simulink model "FmTxRx"  (R2015b)
settings: Solver=VariableStepAuto  StartTime=0.0  StopTime=10.0  RelTol=1e-3
undefined symbols (not defined in the file): SLIF_fc_IM, SLIF_fc_IMDS, SLIF_fc_IMDT, SLIF_fc_LO, SLIF_fc_RF, SLIF_Frame, SLIF_ModIndex, SLIF_PSF_SampPerSym, SLIF_Rsymbol
libraries: dspmathops x8, simrfV2elements x7, dspstat3 x7, simrfV2util1 x6, dspsrcs4 x4, commrflib2 x4, commrandsrc2 x3, commobslib x3, commdigbbndfm2 x3, dspvision x1, dspsnks4 x1
settings Model: Creator=dominikguz  LastModifiedBy=dominikguz

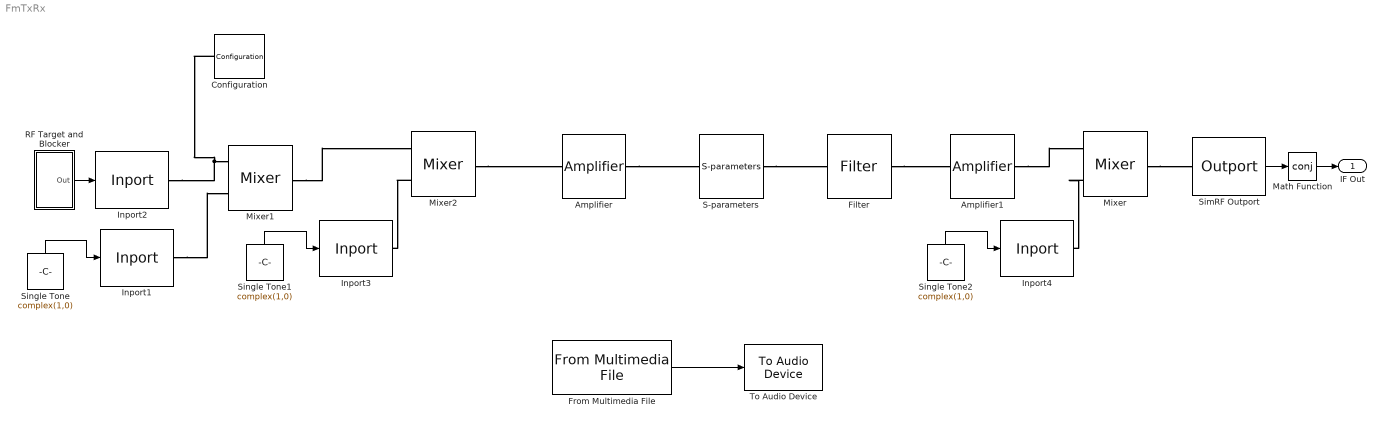
== system FmTxRx ==
  Amplifier : simrfV2elements/Amplifier  classname=amplifier  DataSource=Data file  File=simrfV2_unitygain.s2p  Paramtype=S-parameters  Sparam=[0 0;1 0]  SparamFreq=1e9 Hz  SparamZ0=50  Residues=0  Poles=0  DF={0 0; 1 0}  Source_linear_gain=Available power gain  linear_gain=10 dB  Zin=50  Zout=50  Source_Poly=Even and odd order  Poly_Coeffs=[0 1]  IPType=Output  IP2=inf dBm  IP3=inf dBm  P1dB=inf dBm  Psat=inf dBm  Gcomp=inf dBm  NF=0  InternalGrounding=on  SourceFreq=Extracted from data source  PlotFreq=[1e9:1e6:3e9] Hz  PlotType=X-Y plane  YParam1=S11  YFormat1=Magnitude (decibels)  YParam2=None  YFormat2=Magnitude (decibels)  YOption=Linear  XOption=Linear  SparamRepresentation=Time domain (rationalfit)  FitTol=-40  FitOpt=Fit individually  AutoImpulseLength=on  ImpulseLength=1e-10 s
  Amplifier1 : simrfV2elements/Amplifier  classname=amplifier  DataSource=Data file  File=simrfV2_unitygain.s2p  Paramtype=S-parameters  Sparam=[0 0;1 0]  SparamFreq=1e9 Hz  SparamZ0=50  Residues=0  Poles=0  DF={0 0; 1 0}  Source_linear_gain=Available power gain  linear_gain=10 dB  Zin=50  Zout=50  Source_Poly=Even and odd order  Poly_Coeffs=[0 1]  IPType=Output  IP2=inf dBm  IP3=inf dBm  P1dB=inf dBm  Psat=inf dBm  Gcomp=inf dBm  NF=0  InternalGrounding=on  SourceFreq=Extracted from data source  PlotFreq=[1e9:1e6:3e9] Hz  PlotType=X-Y plane  YParam1=S11  YFormat1=Magnitude (decibels)  YParam2=None  YFormat2=Magnitude (decibels)  YOption=Linear  XOption=Linear  SparamRepresentation=Time domain (rationalfit)  FitTol=-40  FitOpt=Fit individually  AutoImpulseLength=on  ImpulseLength=1e-10 s
  Configuration : simrfV2util1/Configuration  AutoFreq=on  Tones=[] Hz  Harmonics=[]  NormalizeCarrierPower=on  SolverType=Auto  StepSize=1e-6 s  AddNoise=on  Temperature=290.0 K  SolverDelFlag=0
  Filter : simrfV2elements/Filter  classname=filter  DesignMethod=Butterworth  ResponseType=Lowpass  Implementation=LC Tee  UseFilterOrder=on  FilterOrder=3  PassFreq_lp=1 GHz  PassFreq_hp=2 GHz  PassFreq_bp=[2 3] GHz  PassFreq_bs=[1 4] GHz  PassAtten=10*log10(2)  StopFreq_lp=2 GHz  StopFreq_hp=1 GHz  StopFreq_bp=[1.5 3.5] GHz  StopFreq_bs=[2.1 2.9] GHz  StopAtten=40  Rsrc=50  Rload=50  InternalGrounding=on  PlotFuncLeft=Voltage transfer  PlotLeftForm=Magnitude (decibels)  PlotRightOnVT=None  PlotRightNoTD=None  PlotRightNoGD=None  PlotRightNoIR=None  PlotRightNoSR=None  PlotRightForm=Magnitude (decibels)  FreqPoints=logspace(0,10,101)  Freq_unit=Hz  TimePoints=linspace(0,1,1e6+1)  Time_unit=s  XaxisScale=Linear  YaxisScale=Linear
  From Multimedia File : dspvision/From Multimedia File  inputFilename=speech_dft.mp3  loop=on  numPlays=inf  outputStreams=Audio only  videoDataType=single  audioDataType=double  inheritSampleTime=on  userDefinedSampleTime=1/30  noAudioOutput=off  isIntensityVideo=off  fourcc=RGB  colorVideoFormat=Separate color signals  outputEOF=off  dataOrg=Column-major  audioFrameSize=1024  computeAudioFrameSize=off  outSamplingMode=Sample based
  Inport1 : simrfV2util1/Inport  SimulinkInputSignalType=Ideal voltage  CarrierFreq=[SLIF_fc_LO] Hz  ZS=0  InternalGrounding=on
  Inport2 : simrfV2util1/Inport  SimulinkInputSignalType=Ideal voltage  CarrierFreq=[SLIF_fc_RF,SLIF_fc_IM,SLIF_fc_IMDS,SLIF_fc_IMDT] Hz  ZS=0  InternalGrounding=on
  Inport3 : simrfV2util1/Inport  SimulinkInputSignalType=Ideal voltage  CarrierFreq=[SLIF_fc_LO] Hz  ZS=0  InternalGrounding=on
  Inport4 : simrfV2util1/Inport  SimulinkInputSignalType=Ideal voltage  CarrierFreq=[SLIF_fc_LO] Hz  ZS=0  InternalGrounding=on
  Math Function : Math  Operator=conj  SaturateOnIntegerOverflow=on
  Mixer : simrfV2elements/Mixer  classname=mixer  Source_linear_gain=Available power gain  linear_gain=0 dB  Zin=50  Zout=50  ZLO=inf  Source_Poly=Even and odd order  Poly_Coeffs=[0 1]  IPType=Output  IP2=Inf dBm  IP3=Inf dBm  P1dB=Inf dBm  Psat=Inf dBm  Gcomp=Inf dBm  NF=0  InternalGrounding=on
  Mixer1 : simrfV2elements/Mixer  classname=mixer  Source_linear_gain=Available power gain  linear_gain=0 dB  Zin=50  Zout=50  ZLO=inf  Source_Poly=Even and odd order  Poly_Coeffs=[0 1]  IPType=Output  IP2=Inf dBm  IP3=Inf dBm  P1dB=Inf dBm  Psat=Inf dBm  Gcomp=Inf dBm  NF=0  InternalGrounding=on
  Mixer2 : simrfV2elements/Mixer  classname=mixer  Source_linear_gain=Available power gain  linear_gain=0 dB  Zin=50  Zout=50  ZLO=inf  Source_Poly=Even and odd order  Poly_Coeffs=[0 1]  IPType=Output  IP2=Inf dBm  IP3=Inf dBm  P1dB=Inf dBm  Psat=Inf dBm  Gcomp=Inf dBm  NF=0  InternalGrounding=on
  RF Target and Blocker : Subsystem
  S-parameters : simrfV2elements/S-parameters  classname=sparam_element  DataSource=Data file  File=simrfV2_unitygain.s2p  Paramtype=S-parameters  Sparam=[0 0;1 0]  SparamFreq=1e9 Hz  SparamZ0=50  Residues=0  Poles=0  DF={0 0; 1 0}  FitOpt=Share all poles  FitTol=-40  SourceFreq=Extracted from data source  PlotFreq=[1e9:1e6:3e9] Hz  PlotType=X-Y plane  YParam1=S11  YFormat1=Magnitude (decibels)  YParam2=None  YFormat2=Magnitude (decibels)  YOption=Linear  XOption=Linear  AddNoise=off  InternalGrounding=on  SparamRepresentation=Time domain (rationalfit)  AutoImpulseLength=on  ImpulseLength=1e-10 s
  SimRF Outport : simrfV2util1/Outport  SensorType=Ideal voltage  OutputFormat=Complex Baseband  CarrierFreq=SLIF_fc_IF Hz  ZL=Inf  InternalGrounding=on  StepSize=-1 s  AutoStep=off
  Single Tone : Constant  Value=complex(1,0)
  Single Tone1 : Constant  Value=complex(1,0)
  Single Tone2 : Constant  Value=complex(1,0)
  To Audio Device : dspsnks4/To Audio Device  deviceName=Default  inheritSampleRate=on  sampleRate=44100  deviceDatatype=Determine from input data type  autoBufferSize=on  bufferSize=4096  queueDuration=1.0  defaultOutputChannelMapping=on  outputChannelMapping=1:2  outputNumUnderrunSamples=off
  IF Out : Outport
  wires:
  From Multimedia File/1 -> To Audio Device/1
  SimRF Outport/1 -> Math Function/1
  Math Function/1 -> IF Out/1
  RF Target and Blocker/1(Out) -> Inport2/1
  Single Tone/1 -> Inport1/1
  Single Tone1/1 -> Inport3/1
  Single Tone2/1 -> Inport4/1
  connections:
  Filter/RConn1 -- Amplifier1/LConn1
  S-parameters/RConn1 -- Filter/LConn1
  Amplifier/RConn1 -- S-parameters/LConn1
  Mixer2/RConn1 -- Amplifier/LConn1
  Mixer1/RConn1 -- Mixer2/LConn1
  Amplifier1/RConn1 -- Mixer/LConn1
  Configuration/LConn1 -- Inport2/RConn1 -- Mixer1/LConn1
  Mixer/RConn1 -- SimRF Outport/LConn1
  Inport1/RConn1 -- Mixer1/LConn2
  Mixer2/LConn2 -- Inport3/RConn1
  Mixer/LConn2 -- Inport4/RConn1

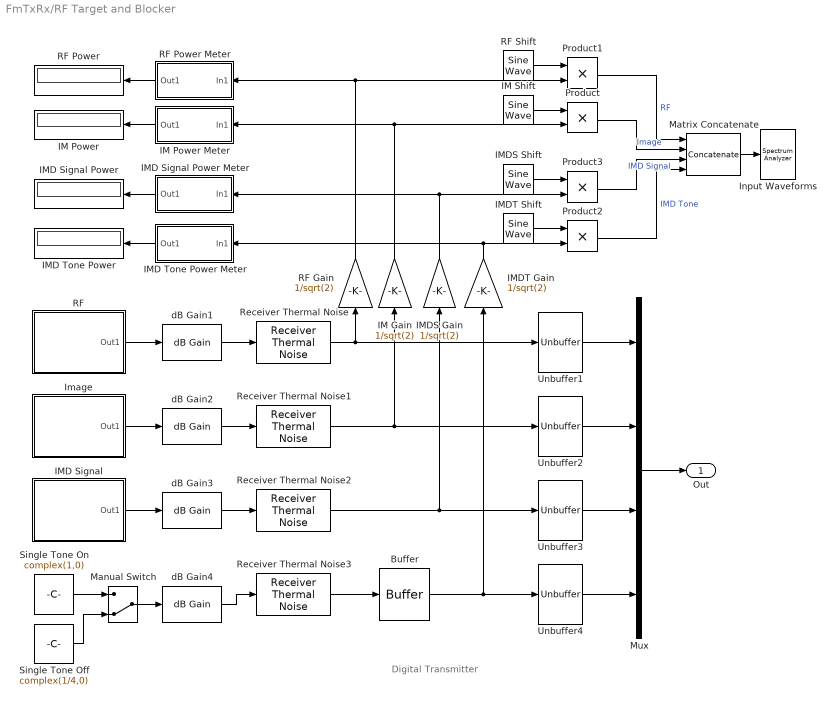
== system FmTxRx/RF Target and Blocker ==
  note: Digital Transmitter
  Buffer : Buffer  N=SLIF_PSF_SampPerSym*SLIF_Frame  TreatMby1Signals=One channel
  IM Gain : Gain  Gain=1/sqrt(2)
  IM Power : Display
  IM Power Meter : Subsystem
  IM Shift : dspsrcs4/Sine Wave  Amplitude=2  Frequency=SLIF_fc_LO-SLIF_fc_RF  Phase=0  SampleMode=Discrete  OutComplex=Complex  CompMethod=Trigonometric fcn  TableSize=Speed  SampleTime=1/(SLIF_Rsymbol*SLIF_PSF_SampPerSym)  SamplesPerFrame=SLIF_PSF_SampPerSym*SLIF_Frame  ResetState=Restart at time zero  OutputFrames=on  dataType=double  wordLen=16  udDataType=sfix(16)  fracBitsMode=Best precision  numFracBits=15  OutDataTypeStr=double  LastOutDataTypeStr=double
  IMD Signal : Subsystem
  IMD Signal Power : Display
  IMD Signal Power Meter : Subsystem
  IMD Tone Power : Display
  IMD Tone Power Meter : Subsystem
  IMDS Gain : Gain  Gain=1/sqrt(2)
  IMDS Shift : dspsrcs4/Sine Wave  Amplitude=2  Frequency=SLIF_fc_IMDS-SLIF_fc_RF  Phase=0  SampleMode=Discrete  OutComplex=Complex  CompMethod=Trigonometric fcn  TableSize=Speed  SampleTime=1/(SLIF_Rsymbol*SLIF_PSF_SampPerSym)  SamplesPerFrame=SLIF_PSF_SampPerSym*SLIF_Frame  ResetState=Restart at time zero  OutputFrames=on  dataType=double  wordLen=16  udDataType=sfix(16)  fracBitsMode=Best precision  numFracBits=15  OutDataTypeStr=double  LastOutDataTypeStr=double
  IMDT Gain : Gain  Gain=1/sqrt(2)
  IMDT Shift : dspsrcs4/Sine Wave  Amplitude=2  Frequency=SLIF_fc_IMDT-SLIF_fc_RF  Phase=0  SampleMode=Discrete  OutComplex=Complex  CompMethod=Trigonometric fcn  TableSize=Speed  SampleTime=1/(SLIF_Rsymbol*SLIF_PSF_SampPerSym)  SamplesPerFrame=SLIF_PSF_SampPerSym*SLIF_Frame  ResetState=Restart at time zero  OutputFrames=on  dataType=double  wordLen=16  udDataType=sfix(16)  fracBitsMode=Best precision  numFracBits=15  OutDataTypeStr=double  LastOutDataTypeStr=double
  Image : Subsystem
  Input Waveforms : SpectrumAnalyzer
  Manual Switch : ManualSwitch  CurrentSetting=0
  Matrix Concatenate : Concatenate  NumInputs=4  Mode=Multidimensional array  ConcatenateDimension=2
  Mux : Mux
  Product{,1..3} (4 alike) : Product  RndMeth=Zero
  RF : Subsystem
  RF Gain : Gain  Gain=1/sqrt(2)
  RF Power : Display
  RF Power Meter : Subsystem
  RF Shift : dspsrcs4/Sine Wave  Amplitude=2  Frequency=0  Phase=0  SampleMode=Discrete  OutComplex=Complex  CompMethod=Trigonometric fcn  TableSize=Speed  SampleTime=1/(SLIF_Rsymbol*SLIF_PSF_SampPerSym)  SamplesPerFrame=SLIF_PSF_SampPerSym*SLIF_Frame  ResetState=Restart at time zero  OutputFrames=on  dataType=double  wordLen=16  udDataType=sfix(16)  fracBitsMode=Best precision  numFracBits=15  OutDataTypeStr=double  LastOutDataTypeStr=double
  Receiver Thermal Noise{,1..3} (4 alike) : commrflib2/Receiver Thermal Noise  method=Noise temperature  ntemp=293  nfigure=3.01  nfactor=2  seed=67987
  Single Tone Off : Constant  Value=complex(1/4,0)
  Single Tone On : Constant  Value=complex(1,0)
  Unbuffer{1..4} (4 alike) : Unbuffer  SampleBasedProcessing=Same as frame based
  dB Gain1 : dspmathops/dB Gain  dB=-97  intype=Amplitude
  dB Gain2 : dspmathops/dB Gain  dB=-67  intype=Amplitude
  dB Gain3 : dspmathops/dB Gain  dB=-60  intype=Amplitude
  dB Gain4 : dspmathops/dB Gain  dB=-60  intype=Amplitude
  Out : Outport
  wires:
  Mux/1 -> Out/1
  RF Power Meter/1(Out1) -> RF Power/1
  IM Power Meter/1(Out1) -> IM Power/1
  Matrix Concatenate/1 -> Input Waveforms/1
  Image/1(Out1) -> dB Gain2/1
  RF/1(Out1) -> dB Gain1/1
  dB Gain1/1 -> Receiver Thermal Noise/1
  Receiver Thermal Noise/1 -> Unbuffer1/1, RF Gain/1
  dB Gain2/1 -> Receiver Thermal Noise1/1
  Receiver Thermal Noise1/1 -> Unbuffer2/1, IM Gain/1
  IM Shift/1 -> Product/1
  RF Shift/1 -> Product1/1
  Product1/1 -> Matrix Concatenate/1  "RF"
  IMD Signal/1(Out1) -> dB Gain3/1
  dB Gain3/1 -> Receiver Thermal Noise2/1
  Receiver Thermal Noise2/1 -> Unbuffer3/1, IMDS Gain/1
  IMD Signal Power Meter/1(Out1) -> IMD Signal Power/1
  dB Gain4/1 -> Receiver Thermal Noise3/1
  Receiver Thermal Noise3/1 -> Buffer/1
  IMD Tone Power Meter/1(Out1) -> IMD Tone Power/1
  IMDS Shift/1 -> Product3/1
  IMDT Shift/1 -> Product2/1
  Product3/1 -> Matrix Concatenate/3  "IMD Signal"
  Product2/1 -> Matrix Concatenate/4  "IMD Tone"
  Single Tone On/1 -> Manual Switch/1
  Single Tone Off/1 -> Manual Switch/2
  Manual Switch/1 -> dB Gain4/1
  Unbuffer4/1 -> Mux/4
  Unbuffer3/1 -> Mux/3
  Unbuffer2/1 -> Mux/2
  Unbuffer1/1 -> Mux/1
  Product/1 -> Matrix Concatenate/2  "Image"
  RF Gain/1 -> RF Power Meter/1(In1), Product1/2
  IM Gain/1 -> Product/2, IM Power Meter/1(In1)
  IMDS Gain/1 -> IMD Signal Power Meter/1(In1), Product3/2
  IMDT Gain/1 -> Product2/2, IMD Tone Power Meter/1(In1)
  Buffer/1 -> Unbuffer4/1, IMDT Gain/1

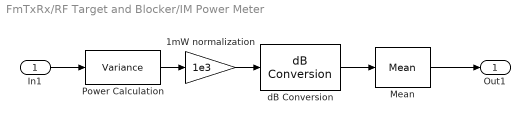
== system FmTxRx/RF Target and Blocker/IM Power Meter ==
  In1 : Inport
  1mW normalization : Gain  Gain=1e3
  Mean : dspstat3/Mean  run=off  reset_popup=None  InputProcessing=Columns as channels (frame based)  directionMode=Each column  dimension=1  roiEnable=off  roiType=Rectangles  roiPortion=Entire ROI  roiOutput=Individual statistics for each ROI  roiFlag=off  outputDataTypeStr=Inherit: Same as accumulator  outputLastDataTypeStr=Inherit: Same as accumulator  outputMin=[]  outputMax=[]  roundingMode=Floor  overflowMode=off
  Power Calculation : dspstat3/Variance  run=on  reset_popup=None  InputProcessing=Columns as channels (frame based)  directionMode=Each column  dimension=1  roiEnable=off  roiType=Rectangles  roiPortion=Entire ROI  roiOutput=Individual statistics for each ROI  roiFlag=off  roundingMode=Floor  overflowMode=off
  dB Conversion : dspmathops/dB Conversion  dBtype=dB  intype=Power  R=1  fuzz=on
  Out1 : Outport
  wires:
  Power Calculation/1 -> 1mW normalization/1
  1mW normalization/1 -> dB Conversion/1
  In1/1 -> Power Calculation/1
  dB Conversion/1 -> Mean/1
  Mean/1 -> Out1/1

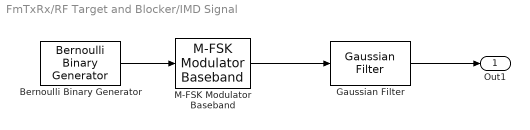
== system FmTxRx/RF Target and Blocker/IMD Signal ==
  Bernoulli Binary Generator : commrandsrc2/Bernoulli Binary Generator  P=0.5  seed=31  Ts=1/SLIF_Rsymbol  frameBased=on  sampPerFrame=SLIF_Frame  orient=off  outDataType=double
  Gaussian Filter : commobslib/Gaussian Filter  N=SLIF_PSF_SampPerSym  BT=SLIF_PSF_BT  D=1  sampMode=Frame-based  normMode=Sum of coefficients  filterGain=1  checkCoeff=off  variableName=gaussFilt  launchFVT=off  roundingMode=Floor  overflowMode=off  InputProcessing=Columns as channels (frame based)
  M-FSK Modulator Baseband : commdigbbndfm2/M-FSK Modulator Baseband  M=2  InType=Integer  Enc=Binary  freqSep=SLIF_ModIndex*SLIF_Rsymbol  phaseType=Continuous  numSamp=SLIF_PSF_SampPerSym  RateOptions=Enforce single-rate processing  outDataType=double
  Out1 : Outport
  wires:
  M-FSK Modulator Baseband/1 -> Gaussian Filter/1
  Bernoulli Binary Generator/1 -> M-FSK Modulator Baseband/1
  Gaussian Filter/1 -> Out1/1

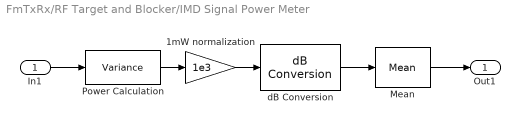
== system FmTxRx/RF Target and Blocker/IMD Signal Power Meter ==
  In1 : Inport
  1mW normalization : Gain  Gain=1e3
  Mean : dspstat3/Mean  run=off  reset_popup=None  InputProcessing=Columns as channels (frame based)  directionMode=Each column  dimension=1  roiEnable=off  roiType=Rectangles  roiPortion=Entire ROI  roiOutput=Individual statistics for each ROI  roiFlag=off  outputDataTypeStr=Inherit: Same as accumulator  outputLastDataTypeStr=Inherit: Same as accumulator  outputMin=[]  outputMax=[]  roundingMode=Floor  overflowMode=off
  Power Calculation : dspstat3/Variance  run=on  reset_popup=None  InputProcessing=Columns as channels (frame based)  directionMode=Each column  dimension=1  roiEnable=off  roiType=Rectangles  roiPortion=Entire ROI  roiOutput=Individual statistics for each ROI  roiFlag=off  roundingMode=Floor  overflowMode=off
  dB Conversion : dspmathops/dB Conversion  dBtype=dB  intype=Power  R=1  fuzz=on
  Out1 : Outport
  wires:
  Power Calculation/1 -> 1mW normalization/1
  1mW normalization/1 -> dB Conversion/1
  In1/1 -> Power Calculation/1
  dB Conversion/1 -> Mean/1
  Mean/1 -> Out1/1

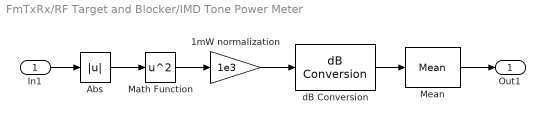
== system FmTxRx/RF Target and Blocker/IMD Tone Power Meter ==
  In1 : Inport
  1mW normalization : Gain  Gain=1e3
  Abs : Abs
  Math Function : Math  Operator=square  SaturateOnIntegerOverflow=on
  Mean : dspstat3/Mean  run=off  reset_popup=None  InputProcessing=Columns as channels (frame based)  directionMode=Each column  dimension=1  roiEnable=off  roiType=Rectangles  roiPortion=Entire ROI  roiOutput=Individual statistics for each ROI  roiFlag=off  outputDataTypeStr=Inherit: Same as accumulator  outputLastDataTypeStr=Inherit: Same as accumulator  outputMin=[]  outputMax=[]  roundingMode=Floor  overflowMode=off
  dB Conversion : dspmathops/dB Conversion  dBtype=dB  intype=Power  R=1  fuzz=on
  Out1 : Outport
  wires:
  Math Function/1 -> 1mW normalization/1
  1mW normalization/1 -> dB Conversion/1
  dB Conversion/1 -> Mean/1
  Abs/1 -> Math Function/1
  In1/1 -> Abs/1
  Mean/1 -> Out1/1

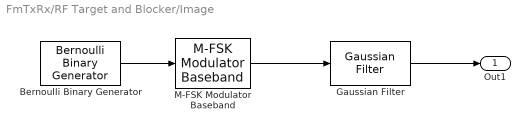
== system FmTxRx/RF Target and Blocker/Image ==
  Bernoulli Binary Generator : commrandsrc2/Bernoulli Binary Generator  P=0.5  seed=21  Ts=1/SLIF_Rsymbol  frameBased=on  sampPerFrame=SLIF_Frame  orient=off  outDataType=double
  Gaussian Filter : commobslib/Gaussian Filter  N=SLIF_PSF_SampPerSym  BT=SLIF_PSF_BT  D=1  sampMode=Frame-based  normMode=Sum of coefficients  filterGain=1  checkCoeff=off  variableName=gaussFilt  launchFVT=off  roundingMode=Floor  overflowMode=off  InputProcessing=Columns as channels (frame based)
  M-FSK Modulator Baseband : commdigbbndfm2/M-FSK Modulator Baseband  M=2  InType=Integer  Enc=Binary  freqSep=SLIF_ModIndex*SLIF_Rsymbol  phaseType=Continuous  numSamp=SLIF_PSF_SampPerSym  RateOptions=Enforce single-rate processing  outDataType=double
  Out1 : Outport
  wires:
  Gaussian Filter/1 -> Out1/1
  Bernoulli Binary Generator/1 -> M-FSK Modulator Baseband/1
  M-FSK Modulator Baseband/1 -> Gaussian Filter/1

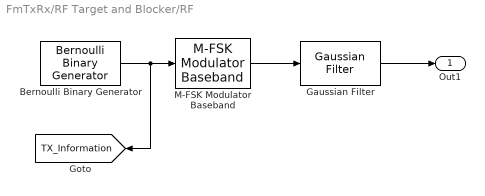
== system FmTxRx/RF Target and Blocker/RF ==
  Bernoulli Binary Generator : commrandsrc2/Bernoulli Binary Generator  P=0.5  seed=11  Ts=1/SLIF_Rsymbol  frameBased=on  sampPerFrame=SLIF_Frame  orient=off  outDataType=double
  Gaussian Filter : commobslib/Gaussian Filter  N=SLIF_PSF_SampPerSym  BT=SLIF_PSF_BT  D=1  sampMode=Frame-based  normMode=Sum of coefficients  filterGain=1  checkCoeff=off  variableName=gaussFilt  launchFVT=off  roundingMode=Floor  overflowMode=off  InputProcessing=Columns as channels (frame based)
  M-FSK Modulator Baseband : commdigbbndfm2/M-FSK Modulator Baseband  M=2  InType=Integer  Enc=Binary  freqSep=SLIF_ModIndex*SLIF_Rsymbol  phaseType=Continuous  numSamp=SLIF_PSF_SampPerSym  RateOptions=Enforce single-rate processing  outDataType=double
  Out1 : Outport
  tag scope: TX_Information=global
  wires:
  M-FSK Modulator Baseband/1 -> Gaussian Filter/1
  Bernoulli Binary Generator/1 -> [TX_Information], M-FSK Modulator Baseband/1
  Gaussian Filter/1 -> Out1/1

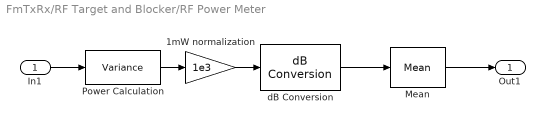
== system FmTxRx/RF Target and Blocker/RF Power Meter ==
  In1 : Inport
  1mW normalization : Gain  Gain=1e3
  Mean : dspstat3/Mean  run=off  reset_popup=None  InputProcessing=Columns as channels (frame based)  directionMode=Each column  dimension=1  roiEnable=off  roiType=Rectangles  roiPortion=Entire ROI  roiOutput=Individual statistics for each ROI  roiFlag=off  outputDataTypeStr=Inherit: Same as accumulator  outputLastDataTypeStr=Inherit: Same as accumulator  outputMin=[]  outputMax=[]  roundingMode=Floor  overflowMode=off
  Power Calculation : dspstat3/Variance  run=on  reset_popup=None  InputProcessing=Columns as channels (frame based)  directionMode=Each column  dimension=1  roiEnable=off  roiType=Rectangles  roiPortion=Entire ROI  roiOutput=Individual statistics for each ROI  roiFlag=off  roundingMode=Floor  overflowMode=off
  dB Conversion : dspmathops/dB Conversion  dBtype=dB  intype=Power  R=1  fuzz=on
  Out1 : Outport
  wires:
  Power Calculation/1 -> 1mW normalization/1
  1mW normalization/1 -> dB Conversion/1
  In1/1 -> Power Calculation/1
  dB Conversion/1 -> Mean/1
  Mean/1 -> Out1/1
